simulink model "bpsk_13_frequency_noise"  (R2018a)
settings: Solver=VariableStepAuto  StartTime=0.0  StopTime=10.0  RelTol=1e-3
libraries: simulink x1, commrandsrc3 x1, dsparch4 x1
settings Model: Creator=hp  LastModifiedBy=hp

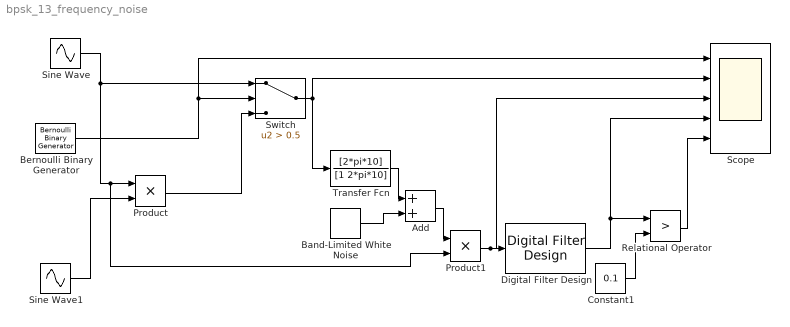
== system bpsk_13_frequency_noise ==
  Add : Sum
  Band-Limited White Noise : simulink/Sources/Band-Limited White Noise  Cov=[0.002]  Ts=0.1  seed=[23341]
  Bernoulli Binary Generator : commrandsrc3/Bernoulli Binary Generator  ProbabilityOfZero=0.5  SeedSource=Auto  Seed=0  SampleTime=1  SamplesPerFrame=1  OutputDataType=double  SimulateUsing=Interpreted execution
  Constant1 : Constant  Value=0.1
  Digital Filter Design : dsparch4/Digital Filter Design  mwdsp_browser_bugfix_var=off
  Product : Product
  Product1 : Product
  Relational Operator : RelationalOperator  Operator=>  OutDataTypeStr=boolean  RndMeth=Simplest
  Scope : Scope  NumInputPorts=5
  Sine Wave : Sin  Amplitude=2  Frequency=2*pi*13  SampleTime=0.01
  Sine Wave1 : Sin  Amplitude=2  Frequency=2*pi*13  Phase=180  SampleTime=0.01
  Switch : Switch  Criteria=u2 > Threshold  Threshold=0.5
  Transfer Fcn : TransferFcn  Numerator=[2*pi*10]  Denominator=[1 2*pi*10]
  wires:
  Sine Wave/1 -> Product1/2, Product/1, Switch/1
  Digital Filter Design/1 -> Scope/4, Relational Operator/1
  Product1/1 -> Scope/3, Digital Filter Design/1
  Sine Wave1/1 -> Product/2
  Bernoulli Binary Generator/1 -> Scope/1, Switch/2
  Relational Operator/1 -> Scope/5
  Constant1/1 -> Relational Operator/2
  Switch/1 -> Transfer Fcn/1, Scope/2
  Product/1 -> Switch/3
  Transfer Fcn/1 -> Add/1
  Band-Limited White Noise/1 -> Add/2
  Add/1 -> Product1/1
